simulink model "amr_industrial_supervisor"  (R2025b)
settings: Solver=FixedStepDiscrete  StartTime=0.0  StopTime=22  FixedStep=0.1  RelTol=1e-3
settings Model: Creator=leeyj  LastModifiedBy=leeyj

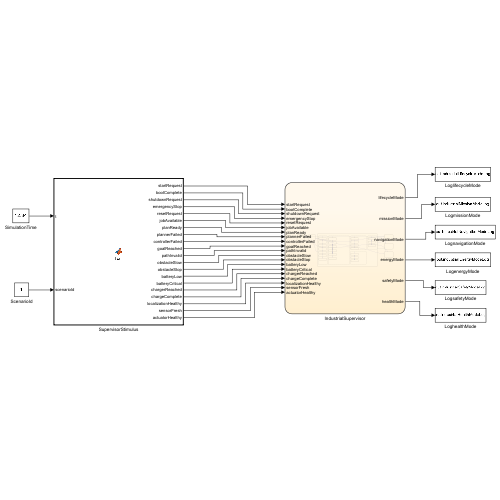
[thumbnail: Simulink's stored preview of the top-level diagram]
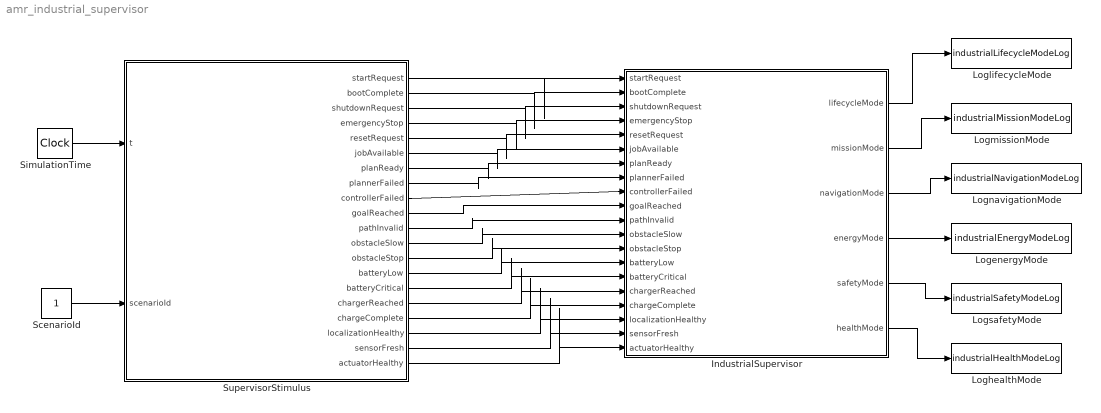
== system amr_industrial_supervisor ==
  IndustrialSupervisor : Stateflow chart  TreatAsAtomicUnit=on
  LogenergyMode : ToWorkspace  VariableName=industrialEnergyModeLog  SaveFormat=Timeseries  SampleTime=-1
  LoghealthMode : ToWorkspace  VariableName=industrialHealthModeLog  SaveFormat=Timeseries  SampleTime=-1
  LoglifecycleMode : ToWorkspace  VariableName=industrialLifecycleModeLog  SaveFormat=Timeseries  SampleTime=-1
  LogmissionMode : ToWorkspace  VariableName=industrialMissionModeLog  SaveFormat=Timeseries  SampleTime=-1
  LognavigationMode : ToWorkspace  VariableName=industrialNavigationModeLog  SaveFormat=Timeseries  SampleTime=-1
  LogsafetyMode : ToWorkspace  VariableName=industrialSafetyModeLog  SaveFormat=Timeseries  SampleTime=-1
  ScenarioId : Constant
  SimulationTime : DigitalClock  SampleTime=0.1
  SupervisorStimulus : MATLAB Function  TreatAsAtomicUnit=on
  wires:
  SupervisorStimulus/5(resetRequest) -> IndustrialSupervisor/5(resetRequest)
  SupervisorStimulus/3(shutdownRequest) -> IndustrialSupervisor/3(shutdownRequest)
  SupervisorStimulus/1(startRequest) -> IndustrialSupervisor/1(startRequest)
  ScenarioId/1 -> SupervisorStimulus/2(scenarioId)
  SimulationTime/1 -> SupervisorStimulus/1(t)
  SupervisorStimulus/6(jobAvailable) -> IndustrialSupervisor/6(jobAvailable)
  SupervisorStimulus/4(emergencyStop) -> IndustrialSupervisor/4(emergencyStop)
  SupervisorStimulus/2(bootComplete) -> IndustrialSupervisor/2(bootComplete)
  SupervisorStimulus/7(planReady) -> IndustrialSupervisor/7(planReady)
  SupervisorStimulus/8(plannerFailed) -> IndustrialSupervisor/8(plannerFailed)
  SupervisorStimulus/9(controllerFailed) -> IndustrialSupervisor/9(controllerFailed)
  SupervisorStimulus/10(goalReached) -> IndustrialSupervisor/10(goalReached)
  SupervisorStimulus/11(pathInvalid) -> IndustrialSupervisor/11(pathInvalid)
  SupervisorStimulus/12(obstacleSlow) -> IndustrialSupervisor/12(obstacleSlow)
  SupervisorStimulus/13(obstacleStop) -> IndustrialSupervisor/13(obstacleStop)
  SupervisorStimulus/14(batteryLow) -> IndustrialSupervisor/14(batteryLow)
  SupervisorStimulus/15(batteryCritical) -> IndustrialSupervisor/15(batteryCritical)
  SupervisorStimulus/16(chargerReached) -> IndustrialSupervisor/16(chargerReached)
  SupervisorStimulus/17(chargeComplete) -> IndustrialSupervisor/17(chargeComplete)
  SupervisorStimulus/18(localizationHealthy) -> IndustrialSupervisor/18(localizationHealthy)
  SupervisorStimulus/19(sensorFresh) -> IndustrialSupervisor/19(sensorFresh)
  SupervisorStimulus/20(actuatorHealthy) -> IndustrialSupervisor/20(actuatorHealthy)
  IndustrialSupervisor/1(lifecycleMode) -> LoglifecycleMode/1
  IndustrialSupervisor/2(missionMode) -> LogmissionMode/1
  IndustrialSupervisor/3(navigationMode) -> LognavigationMode/1
  IndustrialSupervisor/4(energyMode) -> LogenergyMode/1
  IndustrialSupervisor/5(safetyMode) -> LogsafetyMode/1
  IndustrialSupervisor/6(healthMode) -> LoghealthMode/1

== matlab function amr_industrial_supervisor/SupervisorStimulus ==
  data: t input double size=1; startRequest output boolean size=1; scenarioId input double size=1; bootComplete output boolean size=1; shutdownRequest output boolean size=1; emergencyStop output boolean size=1; resetRequest output boolean size=1; jobAvailable output boolean size=1; planReady output boolean size=1; plannerFailed output boolean size=1; controllerFailed output boolean size=1; goalReached output boolean size=1; pathInvalid output boolean size=1; obstacleSlow output boolean size=1; obstacleStop output boolean size=1; batteryLow output boolean size=1; batteryCritical output boolean size=1; chargerReached output boolean size=1; chargeComplete output boolean size=1; localizationHealthy output boolean size=1; sensorFresh output boolean size=1; actuatorHealthy output boolean size=1
function [startRequest,bootComplete,shutdownRequest,emergencyStop,resetRequest,jobAvailable,planReady,plannerFailed,controllerFailed,goalReached,pathInvalid,obstacleSlow,obstacleStop,batteryLow,batteryCritical,chargerReached,chargeComplete,localizationHealthy,sensorFresh,actuatorHealthy] = fcn(t,scenarioId)
startRequest=t>=0.2; bootComplete=t>=1.0; shutdownRequest=false; emergencyStop=false; resetRequest=false;
jobAvailable=t>=2.0 && t<2.3; planReady=true; plannerFailed=false; controllerFailed=false;
goalReached=(t>=8.0&&t<8.3)||(t>=13.0&&t<13.3)||(t>=19.0&&t<19.3); pathInvalid=false;
obstacleSlow=false; obstacleStop=false; batteryLow=false; batteryCritical=false; chargerReached=false; chargeComplete=false;
localizationHealthy=true; sensorFresh=true; actuatorHealthy=true;
if scenarioId==2, obstacleSlow=t>=5&&t<6; obstacleStop=t>=6&&t<8; resetRequest=t>=8; pathInvalid=t>=8&&t<8.3; end
if scenarioId==3, batteryLow=t>=5&&t<15; batteryCritical=t>=7&&t<15; chargerReached=t>=10; chargeComplete=t>=15; end
if scenarioId==4, sensorFresh=~(t>=5&&t<9); localizationHealthy=~(t>=5&&t<9); actuatorHealthy=t<12; resetRequest=t>=16; end
if scenarioId==5, emergencyStop=t>=6&&t<9; resetRequest=t>=9.5; end

== stateflow chart amr_industrial_supervisor/IndustrialSupervisor ==
  state Operational
    entry,during:
    lifecycleMode = uint8(2);
    state MissionRegion [parallel]
      settings: executionOrder=1
      state Idle
        entry,during:
        missionMode = uint8(0);
      state AcceptJob
        entry,during:
        missionMode = uint8(1);
      state NavigatePickup
        entry,during:
        missionMode = uint8(2);
      state Loading
        entry,during:
        missionMode = uint8(3);
      state NavigateDropoff
        entry,during:
        missionMode = uint8(4);
      state Unloading
        entry,during:
        missionMode = uint8(5);
      state ReturnHome
        entry,during:
        missionMode = uint8(6);
      (default) -> Idle
      Idle -> AcceptJob : [jobAvailable]
      ReturnHome -> Idle : [goalReached]
      AcceptJob -> NavigatePickup : after(0.5,sec)
      NavigatePickup -> Loading : [goalReached]
      Loading -> NavigateDropoff : after(1,sec)
      NavigateDropoff -> Unloading : [goalReached]
      Unloading -> ReturnHome : after(1,sec)
    state NavigationRegion [parallel]
      settings: executionOrder=2
      state NavIdle
        entry,during:
        navigationMode = uint8(0);
      state Planning
        entry,during:
        navigationMode = uint8(1);
      state Tracking
        entry,during:
        navigationMode = uint8(2);
      state Replanning
        entry,during:
        navigationMode = uint8(3);
      state Recovery
        entry,during:
        navigationMode = uint8(4);
      state NavFailed
        entry,during:
        navigationMode = uint8(5);
      (default) -> NavIdle
      Tracking -> NavIdle [order 3] : [goalReached]
      NavIdle -> Planning : [missionMode == uint8(2) || missionMode == uint8(4) || missionMode == uint8(6)]
      Planning -> Tracking [order 1] : [planReady]
      Planning -> Recovery [order 2] : [plannerFailed]
      Planning -> Recovery [order 3] : after(3,sec)
      NavFailed -> Planning : [resetRequest]
      Recovery -> Planning [order 1] : [resetRequest]
      Tracking -> Replanning [order 1] : [pathInvalid]
      Tracking -> Recovery [order 2] : [controllerFailed]
      Replanning -> Tracking [order 1] : [planReady]
      Replanning -> Recovery [order 2] : [plannerFailed]
      Replanning -> Recovery [order 3] : after(3,sec)
      Recovery -> NavFailed [order 2] : after(2,sec)
    state EnergyRegion [parallel]
      settings: executionOrder=3
      state EnergyNormal
        entry,during:
        energyMode = uint8(0);
      state EnergyLow
        entry,during:
        energyMode = uint8(1);
      state EnergyCritical
        entry,during:
        energyMode = uint8(2);
      state Charging
        entry,during:
        energyMode = uint8(3);
      (default) -> EnergyNormal
      EnergyLow -> EnergyNormal [order 1] : [~batteryLow]
      Charging -> EnergyNormal : [chargeComplete]
      EnergyNormal -> EnergyLow : [batteryLow]
      EnergyLow -> EnergyCritical [order 2] : [batteryCritical]
      EnergyCritical -> Charging : [chargerReached]
    state SafetyRegion [parallel]
      settings: executionOrder=4
      state Safe
        entry,during:
        safetyMode = uint8(0);
      state Slowdown
        entry,during:
        safetyMode = uint8(1);
      state ProtectiveStop
        entry,during:
        safetyMode = uint8(2);
      (default) -> Safe
      ProtectiveStop -> Safe : [~obstacleStop && resetRequest]
      Slowdown -> Safe [order 2] : [~obstacleSlow && ~obstacleStop]
      Safe -> Slowdown [order 1] : [obstacleSlow]
      Safe -> ProtectiveStop [order 2] : [obstacleStop]
      Slowdown -> ProtectiveStop [order 1] : [obstacleStop]
    state HealthRegion [parallel]
      settings: executionOrder=5
      state Healthy
        entry,during:
        healthMode = uint8(0);
      state Degraded
        entry,during:
        healthMode = uint8(1);
      state HealthFault
        entry,during:
        healthMode = uint8(2);
      (default) -> Healthy
      Degraded -> Healthy [order 1] : [sensorFresh && localizationHealthy && actuatorHealthy]
      Healthy -> Degraded [order 1] : [~sensorFresh || ~localizationHealthy]
      Healthy -> HealthFault [order 2] : [~actuatorHealthy]
      Degraded -> HealthFault [order 2] : [~actuatorHealthy]
      Degraded -> HealthFault [order 3] : after(5,sec)
  state PowerOff
    entry,during:
    lifecycleMode = uint8(0);
    missionMode = uint8(0);
    navigationMode = uint8(0);
    energyMode = uint8(0);
    safetyMode = uint8(0);
    healthMode = uint8(0);
  state Boot
    entry,during:
    lifecycleMode = uint8(1);
    missionMode = uint8(0);
    navigationMode = uint8(0);
    energyMode = uint8(0);
    safetyMode = uint8(0);
    healthMode = uint8(0);
  state ControlledShutdown
    entry,during:
    lifecycleMode = uint8(3);
    missionMode = uint8(0);
    navigationMode = uint8(0);
    energyMode = uint8(0);
    safetyMode = uint8(0);
    healthMode = uint8(0);
  state FaultLatched
    entry,during:
    lifecycleMode = uint8(4);
    missionMode = uint8(0);
    navigationMode = uint8(0);
    energyMode = uint8(0);
    safetyMode = uint8(3);
    healthMode = uint8(2);
  state EmergencyStopLatched
    entry,during:
    lifecycleMode = uint8(5);
    missionMode = uint8(0);
    navigationMode = uint8(0);
    energyMode = uint8(0);
    safetyMode = uint8(3);
    healthMode = uint8(2);
  (default) -> PowerOff
  ControlledShutdown -> PowerOff : after(1,sec)
  PowerOff -> Boot : [startRequest]
  Operational -> ControlledShutdown [order 1] : [shutdownRequest]
  FaultLatched -> Boot : [resetRequest && actuatorHealthy && sensorFresh]
  EmergencyStopLatched -> Boot : [resetRequest && ~emergencyStop]
  Boot -> Operational [order 1] : [bootComplete]
  Boot -> EmergencyStopLatched [order 2] : [emergencyStop]
  Operational -> FaultLatched [order 3] : [healthMode == uint8(2)]
  Operational -> EmergencyStopLatched [order 2] : [emergencyStop]
  data: startRequest input boolean size=1; bootComplete input boolean size=1; shutdownRequest input boolean size=1; emergencyStop input boolean size=1; resetRequest input boolean size=1; jobAvailable input boolean size=1; planReady input boolean size=1; plannerFailed input boolean size=1; controllerFailed input boolean size=1; goalReached input boolean size=1; pathInvalid input boolean size=1; obstacleSlow input boolean size=1; obstacleStop input boolean size=1; batteryLow input boolean size=1; batteryCritical input boolean size=1; chargerReached input boolean size=1; chargeComplete input boolean size=1; localizationHealthy input boolean size=1; sensorFresh input boolean size=1; actuatorHealthy input boolean size=1; lifecycleMode output uint8 size=1; missionMode output uint8 size=1; navigationMode output uint8 size=1; energyMode output uint8 size=1; safetyMode output uint8 size=1; healthMode output uint8 size=1
